simulink model "KF1_Sim"  (R2020a)
settings: Solver=FixedStepAuto  StartTime=0.0  StopTime=100  FixedStep=1e-2  RelTol=1e-3
libraries: commchan3 x5
settings Model: Creator=niran  LastModifiedBy=niranjan.bhujel

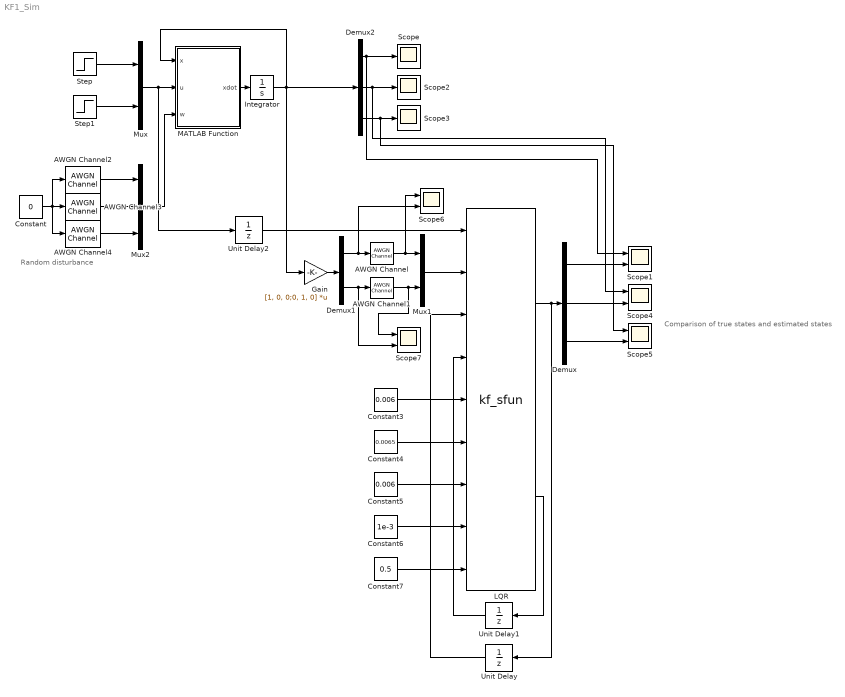
== system KF1_Sim ==
  note: Random disturbance
  note: Comparison of true states and estimated states
  AWGN Channel : commchan3/AWGN Channel  InputProcessing=Columns as channels (frame based)  seed=67  noiseMode=Variance from mask  EbNodB=10  EsNodB=10  SNRdB=10  bitsPerSym=1  Ps=1  Tsym=1  variance=1e-3
  AWGN Channel1 : commchan3/AWGN Channel  InputProcessing=Columns as channels (frame based)  seed=67  noiseMode=Variance from mask  EbNodB=10  EsNodB=10  SNRdB=10  bitsPerSym=1  Ps=1  Tsym=1  variance=0.5
  AWGN Channel2 : commchan3/AWGN Channel  InputProcessing=Columns as channels (frame based)  seed=67  noiseMode=Variance from mask  EbNodB=10  EsNodB=10  SNRdB=1e-4  bitsPerSym=1  Ps=1  Tsym=1  variance=1e-2
  AWGN Channel3 : commchan3/AWGN Channel  InputProcessing=Columns as channels (frame based)  seed=67  noiseMode=Variance from mask  EbNodB=10  EsNodB=10  SNRdB=1e-4  bitsPerSym=1  Ps=1  Tsym=1  variance=0.5
  AWGN Channel4 : commchan3/AWGN Channel  InputProcessing=Columns as channels (frame based)  seed=67  noiseMode=Variance from mask  EbNodB=10  EsNodB=10  SNRdB=1e-4  bitsPerSym=1  Ps=1  Tsym=1  variance=0.1
  Constant : Constant  Value=0
  Constant3 : Constant  Value=0.006
  Constant4 : Constant  Value=0.0065
  Constant5 : Constant  Value=0.006
  Constant6 : Constant  Value=1e-3
  Constant7 : Constant  Value=0.5
  Demux : Demux  Outputs=3
  Demux1 : Demux  Outputs=2
  Demux2 : Demux  Outputs=3
  Gain : Gain  Gain=[1, 0, 0;0, 1, 0]  Multiplication=Matrix(K*u)
  Integrator : Integrator
  LQR : S-Function  InitFcn=try, set_param(gcb,'FunctionName','kf_sfun'), end  FunctionName=kf_sfun  SFunctionModules=kf_sfun_wrapper KF_code KF_code_Call  SFunctionDeploymentMode=off  EnableBusSupport=off  mask(S-Function Builder){}
      mask help: Simulink:masks:SFunctionBuilder_MD
      mask init:
      | val = [[.9  0.75 0.75 1 1 .9 .9 1]',[1 1 0.75 0.75 .9 .9 1 .9]'];try , sys = get_param(gcb,'SfunBuilderFcnName');if isempty(sys), sys = get_param(gcb,'FunctionName'); end,catch, sys = get_param(gcb,'FunctionName'); end
      settings: CopyFcn=set_param(gcbh,'LinkStatus','none')  PreSaveFcn=try, set_param(gcb,'FunctionName','kf_sfun'), end  OpenFcn=sfunctionwizard(gcbh)
      mask Display:
      | plot(val(:,1),val(:,2))
      | disp(sys)
      | port_label('input',1,'u')
      | port_label('input',2,'y')
      | port_label('input',3,'xhatp')
      | port_label('input',4,'Pkp')
      | port_label('input',5,'Q11')
      | port_label('input',6,'Q22')
      | port_label('input',7,'Q33')
      | port_label('input',8,'R11')
      | port_label('input',9,'R22')
      | port_label('output',1,'xhat')
      | port_label('output',2,'Phat')
  MATLAB Function : MATLAB Function  TreatAsAtomicUnit=on
  Mux : Mux  Inputs=2
  Mux1 : Mux  Inputs=2
  Mux2 : Mux  Inputs=3
  Scope : Scope
  Scope{1,4..7} (5 alike) : Scope  NumInputPorts=2
  Scope2 : Scope
  Scope3 : Scope
  Step : Step  Time=50  Before=1  After=2  SampleTime=0
  Step1 : Step  Time=75  Before=0.75  After=1.2  SampleTime=0
  Unit Delay : UnitDelay  InitialCondition=zeros(3, 1)  SampleTime=0.1  HasFrameUpgradeWarning=on
  Unit Delay1 : UnitDelay  InitialCondition=reshape(diag([5, 5, 5]), [9, 1])  SampleTime=0.1  HasFrameUpgradeWarning=on
  Unit Delay2 : UnitDelay  InitialCondition=[0;0]  SampleTime=-1  HasFrameUpgradeWarning=on
  wires:
  Constant3/1 -> LQR/5
  Constant4/1 -> LQR/6
  Constant5/1 -> LQR/7
  LQR/2 -> Unit Delay1/1
  MATLAB Function/1(xdot) -> Integrator/1
  Integrator/1 -> Demux2/1, Gain/1, MATLAB Function/1(x)
  Demux2/1 -> Scope1/1, Scope/1
  Demux2/2 -> Scope4/1, Scope2/1
  Demux2/3 -> Scope3/1, Scope5/1
  Constant6/1 -> LQR/8
  Constant7/1 -> LQR/9
  Mux/1 -> Unit Delay2/1, MATLAB Function/2(u)
  Step/1 -> Mux/1
  Step1/1 -> Mux/2
  LQR/1 -> Unit Delay/1, Demux/1
  Demux/1 -> Scope1/2
  Demux/2 -> Scope4/2
  Demux/3 -> Scope5/2
  Gain/1 -> Demux1/1
  Demux1/1 -> AWGN Channel/1, Scope6/2
  Demux1/2 -> Scope7/2, AWGN Channel1/1
  AWGN Channel/1 -> Scope6/1, Mux1/1
  AWGN Channel1/1 -> Scope7/1, Mux1/2
  Mux1/1 -> LQR/2
  Unit Delay1/1 -> LQR/4
  Unit Delay/1 -> LQR/3
  Constant/1 -> AWGN Channel4/1, AWGN Channel2/1, AWGN Channel3/1
  AWGN Channel3/1 -> Mux2/2
  AWGN Channel2/1 -> Mux2/1
  AWGN Channel4/1 -> Mux2/3
  Mux2/1 -> MATLAB Function/3(w)
  Unit Delay2/1 -> LQR/1

== matlab function KF1_Sim/MATLAB Function ==
  data: x input; u input; xdot output; w input
function xdot = fcn(x, u, w)
    xdot = zeros(3, 1);
    A = [-0.4, 0.1, -2.0;
        0, -0.3, 4.0;
        1.0, 0.0, 0.0];
    B = [1, 1;
        0, 1;
        1, 0];
    
    xdot = A * x + B * u + w;
end
